simulink model "PubIfDecisionTOS_MDL"  (R2020b)
settings: configuration reference "DspaceConfig" (kept outside this file)
PostLoadFcn:
  | if any(exist('dsrtsu_mdlpostloadfcn', 'file') ~= 0), dsrtsu_mdlpostloadfcn('Execute', bdroot); end
InitFcn:
  | , if any(exist('dsmpb_private', 'file') ~= 0), dsmpb_private('dsmpb_mdlclblib', 'Init', bdroot); end,
undefined symbols (not defined in the file or in its folder): C_TOS_ACCEgoRAxletoFbumplength_m, C_TOS_ACCTargetFront_Flag, C_TOS_AEBJAPedObjDxThre_Val, C_TOS_AEBJAPedObjDyThre_Val, C_TOS_AEBJATargetSize_Val, C_TOS_AEBJAVehObjDxThre_Val, C_TOS_AEBJAVehObjDyThre_Val, C_TOS_AEBJuncPedTargetSize_Val, C_TOS_AEBLatObjDxThre_Val, C_TOS_AEBLatPedDyThre_Val, C_TOS_AEBLatTargetSize_Val, C_TOS_AEBLongTargetInEgoFront_Flag, C_TOS_axAbsGround_Parameter, C_TOS_CameraConfirmedFlag, C_TOS_CNsubjWidth, C_TOS_CurrentLaneCoreMinWidth_Val, C_TOS_CutInProb_Val_Zero, C_TOS_CutOutProb_Val_Zero, C_TOS_D2R_Val, C_TOS_DefaultValueObjectToCenterLine_dy, C_TOS_EgoCarWidth_Val, C_TOS_EgoDxRefPoint_m, C_TOS_EgoRAxletoFbumplength_m, C_TOS_HalfWidthVehicle_Con, C_TOS_HWA_CurrentLaneFlag, C_TOS_HWA_LeftLaneFlag, C_TOS_HWA_MovingDir_Vaild, C_TOS_HWA_MovState_Vaild, C_TOS_HWA_RightLaneFlag, C_TOS_LaneLineCourseErrorFront, C_TOS_LaneLineCourseErrorRear, C_TOS_MotorbikeDefaultWidth_m, C_TOS_NumberOfEffectiveTargets, C_TOS_Obj_Age_Val, C_TOS_Objdx_Constraint_Val, C_TOS_ObjectDefaultWidth_m, C_TOS_ObjInCurrentLane_Val, C_TOS_ObjInCurrentLaneValid, C_TOS_ObjInLeftLaneValid, C_TOS_ObjInRightLaneValid, C_TOS_ObjNotInCurrentLane_Val, C_TOS_ObjNotREElementType, C_TOS_ObjPredictDis_dy_ConstantVal_Zeros, C_TOS_ObjToCenterLine_ConstantVal_Zeros, C_TOS_OFMObjIDInvilad_Val, C_TOS_PIL_LatDisCons_Val_zero, C_TOS_PIL_ObjectCutInFlag_b, C_TOS_PIL_ObjectCutOutFlag_b, C_TOS_PIL_ObjLaneProb_al_Val, C_TOS_PP_ObjFusType_FC_Confirm_b, C_TOS_PP_ObjFusType_FC_FR_Confirm_b, C_TOS_PP_ObjFusType_FR_Confirm_b, C_TOS_RE_80BoolDefault_Val, C_TOS_RE_80Single181Default_Val, C_TOS_RE_80Single255Default_Val, C_TOS_RE_80Uint8Default_Val, C_TOS_RE_D2R, C_TOS_RE_D_180_Val, C_TOS_RE_InvalidObjectID_Val, C_TOS_RE_InvalidTargetChainDir_Val ... (+142)
libraries: simulink x1650, TOS_LIB x361, canfdmsglib x14
(part 40 of 69)

== system PubIfDecisionTOS_MDL/TOS_20201112/TOS_2012080320/TOS/LC_LCKie_ELK/TOS_HWA/CurrentLane/HWA_CurrentLane_Target/HWA_CLF_Target_3/HWA_CLR_Target_Default ==
  Action Port : ActionPort  ActionPortLabel=if(u1 ~= 0)
  Constant{1..4,7,12} (6 alike) : Constant  Value=0  OutDataTypeStr=boolean
  HWA_CLR_Target_3_TargeConfirm : Outport
  HWA_CLR_Target_3_MovState_ObserVale : Outport  Port=2
  HWA_CLR_Target_3_ObjType_ObserVale : Outport  Port=3
  HWA_CLR_Target_3_InCurrentLane_Flag_ObserVale : Outport  Port=4
  HWA_CLR_Target_3_TargetMovingDir_ObserVale : Outport  Port=5
  HWA_CLR_Target_3_DyConfirm_ObserVale : Outport  Port=6
  wires:
  Constant4/1 -> HWA_CLR_Target_3_TargeConfirm/1
  Constant1/1 -> HWA_CLR_Target_3_MovState_ObserVale/1
  Constant3/1 -> HWA_CLR_Target_3_ObjType_ObserVale/1
  Constant2/1 -> HWA_CLR_Target_3_InCurrentLane_Flag_ObserVale/1
  Constant12/1 -> HWA_CLR_Target_3_DyConfirm_ObserVale/1
  Constant7/1 -> HWA_CLR_Target_3_TargetMovingDir_ObserVale/1

== system PubIfDecisionTOS_MDL/TOS_20201112/TOS_2012080320/TOS/LC_LCKie_ELK/TOS_HWA/CurrentLane/HWA_Object_PreConfirm/TOS_HWA_CurrentLaneFront_TargPreConfirm/Default ==
  Action Port : ActionPort  ActionPortLabel=else
  Constant{1..10} (10 alike) : Constant  Value=0  OutDataTypeStr=boolean
  TOS_HWA_TargetPre_Filt_Flag : Outport
  TOS_HWA_TargetPre_1_ConditionFlag_ObserVale : Outport  Port=2
  TOS_HWA_TargetPre_FusionTypeFlag_ObserVale : Outport  Port=3
  TOS_HWA_TargetPre_PassedbyTarget_Flag_ObserVale : Outport  Port=4
  TOS_HWA_TargetPre_FenceFlag_ObserVale : Outport  Port=5
  TOS_HWA_TargetPre_ObjType_ObserVale : Outport  Port=6
  TOS_HWA_TargetPre_OverlapThre_Val_ObserVale : Outport  Port=7
  TOS_HWA_TargetPre_SameLane_Flag : Outport  Port=8
  TOS_HWA_TargetPre_2_OverlapThre_ObserVale : Outport  Port=9
  TOS_HWA_TargetPre_3_SameLane_Flag_ObserVale : Outport  Port=10
  wires:
  Constant2/1 -> TOS_HWA_TargetPre_Filt_Flag/1
  Constant9/1 -> TOS_HWA_TargetPre_3_SameLane_Flag_ObserVale/1
  Constant1/1 -> TOS_HWA_TargetPre_1_ConditionFlag_ObserVale/1
  Constant3/1 -> TOS_HWA_TargetPre_FusionTypeFlag_ObserVale/1
  Constant4/1 -> TOS_HWA_TargetPre_PassedbyTarget_Flag_ObserVale/1
  Constant5/1 -> TOS_HWA_TargetPre_FenceFlag_ObserVale/1
  Constant6/1 -> TOS_HWA_TargetPre_ObjType_ObserVale/1
  Constant7/1 -> TOS_HWA_TargetPre_OverlapThre_Val_ObserVale/1
  Constant8/1 -> TOS_HWA_TargetPre_SameLane_Flag/1
  Constant10/1 -> TOS_HWA_TargetPre_2_OverlapThre_ObserVale/1

== system PubIfDecisionTOS_MDL/TOS_20201112/TOS_2012080320/TOS/LC_LCKie_ELK/TOS_HWA/CurrentLane/HWA_Object_PreConfirm/TOS_HWA_CurrentLaneFront_TargPreConfirm/TOS_HWA_CurrentLaneFront_TargPreConfirm ==
  note: 行人、自行车目标过滤
  note: 判断是否为护栏目标
  note: 针对，选中目标后，过滤突然出现的纵向距离更近的单雷达静止目标
  Object_ID : Inport
  PP_ObjFusType_FC_FR_Confirm : Inport  Port=2
  PP_ObjFusType_FR_Confirm : Inport  Port=3
  PP_ObjFusType_FC_Confirm : Inport  Port=4
  Obj_MovingState : Inport  Port=5
  Obj_Dx : Inport  Port=6
  Object_ObstacleProb : Inport  Port=7
  Object_DY : Inport  Port=8
  Object_ObjType : Inport  Port=9
  TOS_TLJ_SameLaneConfirm_Flag : Inport  Port=10
  LM_LR_Line04_fCamValid : Inport  Port=11
  LM_LR_Line05_fCamValid : Inport  Port=12
  LM_LR_Line06_fCamValid : Inport  Port=13
  TOS_HWA_ID_K1 : Inport  Port=14
  TOS_HWA_Dx_K1 : Inport  Port=15
  PIL_OverlapRatio : Inport  Port=16
  PIL_OverlapRatio_K1 : Inport  Port=17
  PIL_OverlapRatio_K2 : Inport  Port=18
  LM_LR_Line04_dDisStart : Inport  Port=19
  LM_LR_Line04_dDisEnd : Inport  Port=20
  LM_LR_Line05_dDisStart : Inport  Port=21
  LM_LR_Line05_dDisEnd : Inport  Port=22
  LM_LR_Line06_dDisStart : Inport  Port=23
  LM_LR_Line06_dDisEnd : Inport  Port=24
  Action Port : ActionPort  ActionPortLabel=if(u1 == 1)
  " " : Subsystem
  Bus Creator : BusCreator  Inputs=24
  Bus Selector1 : BusSelector  OutputSignals=PP_ObjFusType_FR_Confirm,Obj_MovingState,Obj_Dx,TOS_HWA_ID_K1,TOS_HWA_Dx_K1,Object_ID
  Bus Selector2 : BusSelector  OutputSignals=PP_ObjFusType_FC_FR_Confirm,PP_ObjFusType_FC_Confirm,PP_ObjFusType_FR_Confirm
  Bus Selector3 : BusSelector  OutputSignals=PP_ObjFusType_FR_Confirm,Obj_MovingState,Object_ObstacleProb,Object_DY
  Bus Selector4 : BusSelector  OutputSignals=Obj_MovingState,Object_ObjType
  Bus Selector6 : BusSelector  OutputSignals=TOS_TLJ_SameLaneConfirm_Flag
  Compare To Constant2 : simulink/Logic and Bit Operations/Compare To Constant  relop===  const=C_TOS_ACCTargetFront_Flag  OutDataTypeStr=boolean
      settings: AttributesFormatString=C_TOS_ACCTargetFront_Flag = 1
  Logical Operator : Logic  Operator=NOT  AllPortsSameDT=off  OutDataTypeStr=boolean
  Logical Operator1 : Logic  Inputs=5  AllPortsSameDT=off  OutDataTypeStr=boolean
  Logical Operator2 : Logic  Operator=NOT  AllPortsSameDT=off  OutDataTypeStr=boolean
  Logical Operator3 : Logic  Operator=OR  AllPortsSameDT=off  OutDataTypeStr=boolean
  Overlap : Subsystem
  Subsystem : Subsystem
  Subsystem1 : Subsystem
  Subsystem3 : Subsystem
  TOS_HWA_DyConfirm : Subsystem
  TOS_HWA_TargetPre_Filt_Flag : Outport
  TOS_HWA_TargetPre_1_ConditionFlag_ObserVale : Outport  Port=2
  TOS_HWA_TargetPre_FusionTypeFlag_ObserVale : Outport  Port=3
  TOS_HWA_TargetPre_PassedbyTarget_Flag_ObserVale : Outport  Port=4
  TOS_HWA_TargetPre_FenceFlag_ObserVale : Outport  Port=5
  TOS_HWA_TargetPre_ObjType_ObserVale : Outport  Port=6
  TOS_HWA_TargetPre_OverlapThre_Val_ObserVale : Outport  Port=7
  TOS_HWA_TargetPre_SameLane_Flag : Outport  Port=8
  TOS_HWA_TargetPre_2_OverlapThre_ObserVale : Outport  Port=9
  TOS_HWA_TargetPre_3_SameLane_Flag_ObserVale : Outport  Port=10
  wires:
  Subsystem/1(TOS_HWA_TargetPre_TargetFusionTypeFlag) -> [TOS_HWA_TargetPre_FusionTypeFlag_ObserVale], Logical Operator1/1
  Subsystem1/1(TOS_HWA_TargetPre_ObjectPassedbyTarget_Flag) -> Logical Operator/1
  Subsystem3/1(TOS_HWA_TargetPre_FenceFlag) -> Logical Operator2/1
  Logical Operator2/1 -> [TOS_HWA_TargetPre_FenceFlag_ObserVale], Logical Operator1/3
  Logical Operator/1 -> [TOS_HWA_TargetPre_PassedbyTarget_Flag_ObserVale], Logical Operator1/2
  Bus Selector1/6 -> Subsystem1/6(Object_ID)  "<Object_ID>"
  PP_ObjFusType_FR_Confirm/1 -> Bus Creator/3  "PP_ObjFusType_FR_Confirm"
  Bus Selector1/4 -> Subsystem1/4(TOS_HWA_ID_K1)  "<TOS_HWA_ID_K1>"
  Object_ID/1 -> Bus Creator/1  "Object_ID"
  PP_ObjFusType_FC_Confirm/1 -> Bus Creator/4  "PP_ObjFusType_FC_Confirm"
  Bus Selector2/1 -> Subsystem/1(PP_ObjFusType_FC_FR_Confirm)  "<PP_ObjFusType_FC_FR_Confirm>"
  Bus Selector2/3 -> Subsystem/3(PP_ObjFusType_FC_Confirm)  "<PP_ObjFusType_FR_Confirm>"
  Bus Selector1/1 -> Subsystem1/1(FR_Confirm)  "<PP_ObjFusType_FR_Confirm>"
  Bus Selector2/2 -> Subsystem/2(PP_ObjFusType_FR_Confirm)  "<PP_ObjFusType_FC_Confirm>"
  Bus Selector1/5 -> Subsystem1/5(TOS_HWA_Dx_K1)  "<TOS_HWA_Dx_K1>"
  PP_ObjFusType_FC_FR_Confirm/1 -> Bus Creator/2  "PP_ObjFusType_FC_FR_Confirm"
  TOS_HWA_ID_K1/1 -> Bus Creator/14  "TOS_HWA_ID_K1"
  Object_DY/1 -> Bus Creator/8  "Object_DY"
  Bus Selector1/2 -> Subsystem1/2(Obj_MovingState)  "<Obj_MovingState>"
  Bus Selector3/2 -> Subsystem3/2(Obj_MovingState)  "<Obj_MovingState>"
  TOS_HWA_Dx_K1/1 -> Bus Creator/15  "TOS_HWA_Dx_K1"
  Obj_MovingState/1 -> Bus Creator/5  "Obj_MovingState"
  Bus Selector1/3 -> Subsystem1/3(Obj_Dx)  "<Obj_Dx>"
  Object_ObstacleProb/1 -> Bus Creator/7  "Object_ObstacleProb"
  Bus Selector3/3 -> Subsystem3/3(Object_ObstacleProb)  "<Object_ObstacleProb>"
  Bus Selector3/4 -> Subsystem3/4(Object_DY)  "<Object_DY>"
  Bus Selector3/1 -> Subsystem3/1(FR_Confirm)  "<PP_ObjFusType_FR_Confirm>"
  Obj_Dx/1 -> Bus Creator/6  "Obj_Dx"
  Bus Selector4/2 -> " "/2(Object_Type)  "<Object_ObjType>"
  Bus Selector4/1 -> " "/1(object_MovingState)  "<Obj_MovingState>"
  " "/1(TOS_HWA_ObjType) -> [TOS_HWA_TargetPre_ObjType_ObserVale], Logical Operator1/4
  Object_ObjType/1 -> Bus Creator/9  "Object_ObjType"
  [TOS_HWA_TargetPre_FusionTypeFlag_ObserVale] -> TOS_HWA_TargetPre_FusionTypeFlag_ObserVale/1
  [TOS_HWA_TargetPre_PassedbyTarget_Flag_ObserVale] -> TOS_HWA_TargetPre_PassedbyTarget_Flag_ObserVale/1
  [TOS_HWA_TargetPre_FenceFlag_ObserVale] -> TOS_HWA_TargetPre_FenceFlag_ObserVale/1
  [TOS_HWA_TargetPre_ObjType_ObserVale] -> TOS_HWA_TargetPre_ObjType_ObserVale/1
  PIL_OverlapRatio/1 -> Bus Creator/16  "PIL_OverlapRatio"
  TOS_HWA_DyConfirm/1(TOS_HWA_DyConfirm) -> [TOS_HWA_TargetPre_OverlapThre_Val_ObserVale], Logical Operator1/5
  [TOS_HWA_TargetPre_OverlapThre_Val_ObserVale] -> TOS_HWA_TargetPre_OverlapThre_Val_ObserVale/1
  TOS_TLJ_SameLaneConfirm_Flag/1 -> Bus Creator/10  "TOS_TLJ_SameLaneConfirm_Flag"
  Bus Selector6/1 -> Compare To Constant2/1  "<TOS_TLJ_SameLaneConfirm_Flag>"
  Compare To Constant2/1 -> [TOS_HWA_TargetPre_3_SameLane_Flag_ObserVale], Logical Operator3/2
  Logical Operator3/1 -> TOS_HWA_TargetPre_SameLane_Flag/1
  Logical Operator1/1 -> [TOS_HWA_TargetPre_1_ConditionFlag_ObserVale], TOS_HWA_TargetPre_Filt_Flag/1
  [TOS_HWA_TargetPre_2_OverlapThre_ObserVale] -> TOS_HWA_TargetPre_2_OverlapThre_ObserVale/1
  [TOS_HWA_TargetPre_3_SameLane_Flag_ObserVale] -> TOS_HWA_TargetPre_3_SameLane_Flag_ObserVale/1
  [TOS_HWA_TargetPre_1_ConditionFlag_ObserVale] -> TOS_HWA_TargetPre_1_ConditionFlag_ObserVale/1
  PIL_OverlapRatio_K1/1 -> Bus Creator/17  "PIL_OverlapRatio_K1"
  PIL_OverlapRatio_K2/1 -> Bus Creator/18  "PIL_OverlapRatio_K2"
  LM_LR_Line04_fCamValid/1 -> Bus Creator/11  "LM_LR_Line04_fCamValid"
  LM_LR_Line05_fCamValid/1 -> Bus Creator/12  "LM_LR_Line05_fCamValid"
  LM_LR_Line06_fCamValid/1 -> Bus Creator/13  "LM_LR_Line06_fCamValid"
  LM_LR_Line04_dDisStart/1 -> Bus Creator/19  "LM_LR_Line04_dDisStart"
  LM_LR_Line04_dDisEnd/1 -> Bus Creator/20  "LM_LR_Line04_dDisEnd"
  LM_LR_Line05_dDisStart/1 -> Bus Creator/21  "LM_LR_Line05_dDisStart"
  LM_LR_Line05_dDisEnd/1 -> Bus Creator/22  "LM_LR_Line05_dDisEnd"
  LM_LR_Line06_dDisStart/1 -> Bus Creator/23  "LM_LR_Line06_dDisStart"
  LM_LR_Line06_dDisEnd/1 -> Bus Creator/24  "LM_LR_Line06_dDisEnd"
  Bus Creator/1 -> Bus Selector6/1, Overlap/1(LM), TOS_HWA_DyConfirm/1(TOS_HWA_Dy), Bus Selector4/1, Bus Selector3/1, Bus Selector1/1, Bus Selector2/1
  Overlap/1(Overlap) -> [TOS_HWA_TargetPre_2_OverlapThre_ObserVale], Logical Operator3/1

== system PubIfDecisionTOS_MDL/TOS_20201112/TOS_2012080320/TOS/LC_LCKie_ELK/TOS_HWA/CurrentLane/HWA_Object_PreConfirm/TOS_HWA_CurrentLaneFront_TargPreConfirm/TOS_HWA_CurrentLaneRear_TargPreConfirmDefault ==
  Action Port : ActionPort  ActionPortLabel=elseif(u2 == 1)
  Constant{1..10} (10 alike) : Constant  OutDataTypeStr=boolean
  TOS_HWA_TargetPre_Filt_Flag : Outport
  TOS_HWA_TargetPre_1_ConditionFlag_ObserVale : Outport  Port=2
  TOS_HWA_TargetPre_FusionTypeFlag_ObserVale : Outport  Port=3
  TOS_HWA_TargetPre_PassedbyTarget_Flag_ObserVale : Outport  Port=4
  TOS_HWA_TargetPre_FenceFlag_ObserVale : Outport  Port=5
  TOS_HWA_TargetPre_ObjType_ObserVale : Outport  Port=6
  TOS_HWA_TargetPre_OverlapThre_Val_ObserVale : Outport  Port=7
  TOS_HWA_TargetPre_SameLane_Flag : Outport  Port=8
  TOS_HWA_TargetPre_2_OverlapThre_ObserVale : Outport  Port=9
  TOS_HWA_TargetPre_3_SameLane_Flag_ObserVale : Outport  Port=10
  wires:
  Constant10/1 -> TOS_HWA_TargetPre_2_OverlapThre_ObserVale/1
  Constant8/1 -> TOS_HWA_TargetPre_SameLane_Flag/1
  Constant7/1 -> TOS_HWA_TargetPre_OverlapThre_Val_ObserVale/1
  Constant6/1 -> TOS_HWA_TargetPre_ObjType_ObserVale/1
  Constant5/1 -> TOS_HWA_TargetPre_FenceFlag_ObserVale/1
  Constant4/1 -> TOS_HWA_TargetPre_PassedbyTarget_Flag_ObserVale/1
  Constant3/1 -> TOS_HWA_TargetPre_FusionTypeFlag_ObserVale/1
  Constant1/1 -> TOS_HWA_TargetPre_1_ConditionFlag_ObserVale/1
  Constant9/1 -> TOS_HWA_TargetPre_3_SameLane_Flag_ObserVale/1
  Constant2/1 -> TOS_HWA_TargetPre_Filt_Flag/1

== system PubIfDecisionTOS_MDL/TOS_20201112/TOS_2012080320/TOS/LC_LCKie_ELK/TOS_HWA/LeftLane/HWA_Object_PreConfirm/HWA_Object_PreConfirm/Default ==
  Action Port : ActionPort  ActionPortLabel=else
  Constant{2,5..6,8,10} (5 alike) : Constant  Value=0  OutDataTypeStr=boolean
  TOS_HWA_TargetPre_Confirm_Filt_Flag : Outport
  TOS_HWA_TargetPre_FusionTypeFlag_ObserVale : Outport  Port=2
  TOS_HWA_TargetPre_PassedbyTarget_Flag_ObserVale : Outport  Port=3
  TOS_HWA_TargetPre_ObjType_ObserVale : Outport  Port=4
  TOS_HWA_DyConfirm_ObserVale : Outport  Port=5
  wires:
  Constant2/1 -> TOS_HWA_TargetPre_Confirm_Filt_Flag/1
  Constant5/1 -> TOS_HWA_TargetPre_FusionTypeFlag_ObserVale/1
  Constant6/1 -> TOS_HWA_TargetPre_PassedbyTarget_Flag_ObserVale/1
  Constant8/1 -> TOS_HWA_TargetPre_ObjType_ObserVale/1
  Constant10/1 -> TOS_HWA_DyConfirm_ObserVale/1

== system PubIfDecisionTOS_MDL/TOS_20201112/TOS_2012080320/TOS/LC_LCKie_ELK/TOS_HWA/LeftLane/HWA_Object_PreConfirm/HWA_Object_PreConfirm/HWA_Object_PreConfirm ==
  Object_ID : Inport
  PP_ObjFusType_FC_FR_Confirm : Inport  Port=2
  PP_ObjFusType_FR_Confirm : Inport  Port=3
  PP_ObjFusType_FC_Confirm : Inport  Port=4
  Obj_MovingState : Inport  Port=5
  Obj_Dx : Inport  Port=6
  Object_ObstacleProb : Inport  Port=7
  Object_DY : Inport  Port=8
  Object_ObjType : Inport  Port=9
  Action Port : ActionPort  ActionPortLabel=if(u1 == 1)
  " " : Subsystem
  Bus Creator : BusCreator  Inputs=9
  Bus Selector1 : BusSelector  OutputSignals=PP_ObjFusType_FC_Confirm,Obj_MovingState
  Bus Selector2 : BusSelector  OutputSignals=PP_ObjFusType_FC_FR_Confirm,PP_ObjFusType_FC_Confirm,PP_ObjFusType_FR_Confirm
  Bus Selector4 : BusSelector  OutputSignals=Object_ObjType
  Constant1 : Constant  OutDataTypeStr=boolean
  Logical Operator1 : Logic  Inputs=4  AllPortsSameDT=off  OutDataTypeStr=boolean
  Subsystem : Subsystem
  Subsystem1 : Subsystem
  TOS_HWA_DyConfirm : Subsystem
  Terminator : Terminator
  TOS_HWA_TargetPre_Confirm_Filt_Flag : Outport
  TOS_HWA_TargetPre_FusionTypeFlag_ObserVale : Outport  Port=2
  TOS_HWA_TargetPre_PassedbyTarget_Flag_ObserVale : Outport  Port=3
  TOS_HWA_TargetPre_ObjType_ObserVale : Outport  Port=4
  TOS_HWA_DyConfirm_ObserVale : Outport  Port=5
  wires:
  Subsystem/1(TOS_HWA_TargetPre_TargetFusionTypeFlag) -> [TOS_HWA_TargetPre_FusionTypeFlag_ObserVale], Logical Operator1/1
  Subsystem1/1(TOS_HWA_TargetPre_ObjectPassedbyTarget_Flag) -> [TOS_HWA_TargetPre_PassedbyTarget_Flag_ObserVale], Logical Operator1/2
  PP_ObjFusType_FR_Confirm/1 -> Bus Creator/3  "PP_ObjFusType_FR_Confirm"
  Object_ID/1 -> Bus Creator/1  "Object_ID"
  PP_ObjFusType_FC_Confirm/1 -> Bus Creator/4  "PP_ObjFusType_FC_Confirm"
  Bus Selector2/1 -> Subsystem/1(PP_ObjFusType_FC_FR_Confirm)  "<PP_ObjFusType_FC_FR_Confirm>"
  Bus Selector2/3 -> Subsystem/3(PP_ObjFusType_FC_Confirm)  "<PP_ObjFusType_FR_Confirm>"
  Bus Selector1/1 -> Subsystem1/1(PP_ObjFusType_FC_Confirm)  "<PP_ObjFusType_FC_Confirm>"
  Bus Selector2/2 -> Subsystem/2(PP_ObjFusType_FR_Confirm)  "<PP_ObjFusType_FC_Confirm>"
  PP_ObjFusType_FC_FR_Confirm/1 -> Bus Creator/2  "PP_ObjFusType_FC_FR_Confirm"
  Object_DY/1 -> Bus Creator/8  "Object_DY"
  Bus Selector1/2 -> Subsystem1/2(Obj_MovingState)  "<Obj_MovingState>"
  Obj_MovingState/1 -> Bus Creator/5  "Obj_MovingState"
  Object_ObstacleProb/1 -> Bus Creator/7  "Object_ObstacleProb"
  Obj_Dx/1 -> Bus Creator/6  "Obj_Dx"
  Bus Selector4/1 -> " "/1(Object_Type)  "<Object_ObjType>"
  " "/1(TOS_HWA_TargetPre_ObjType) -> Logical Operator1/3, [TOS_HWA_TargetPre_ObjType_ObserVale]
  Object_ObjType/1 -> Bus Creator/9  "Object_ObjType"
  [TOS_HWA_TargetPre_FusionTypeFlag_ObserVale] -> TOS_HWA_TargetPre_FusionTypeFlag_ObserVale/1
  [TOS_HWA_TargetPre_PassedbyTarget_Flag_ObserVale] -> TOS_HWA_TargetPre_PassedbyTarget_Flag_ObserVale/1
  [TOS_HWA_TargetPre_ObjType_ObserVale] -> TOS_HWA_TargetPre_ObjType_ObserVale/1
  Constant1/1 -> Logical Operator1/4, [TOS_HWA_DyConfirm_ObserVale]
  [TOS_HWA_DyConfirm_ObserVale] -> TOS_HWA_DyConfirm_ObserVale/1
  Logical Operator1/1 -> TOS_HWA_TargetPre_Confirm_Filt_Flag/1
  Bus Creator/1 -> TOS_HWA_DyConfirm/1(TOS_HWA_Dy), Bus Selector4/1, Bus Selector1/1, Bus Selector2/1
  TOS_HWA_DyConfirm/1(TOS_HWA_TargetPre_DyConfirm) -> Terminator/1

== system PubIfDecisionTOS_MDL/TOS_20201112/TOS_2012080320/TOS/LC_LCKie_ELK/TOS_HWA/LeftLane/HWA_Object_PreConfirm/HWA_Object_PreConfirm/HWA_Object_PreConfirmDefault1 ==
  Action Port : ActionPort  ActionPortLabel=elseif(u2 == 1)
  Constant{1..5} (5 alike) : Constant  OutDataTypeStr=boolean
  TOS_HWA_TargetPre_Confirm_Filt_Flag : Outport
  TOS_HWA_TargetPre_FusionTypeFlag_ObserVale : Outport  Port=2
  TOS_HWA_TargetPre_PassedbyTarget_Flag_ObserVale : Outport  Port=3
  TOS_HWA_TargetPre_ObjType_ObserVale : Outport  Port=4
  TOS_HWA_DyConfirm_ObserVale : Outport  Port=5
  wires:
  Constant5/1 -> TOS_HWA_DyConfirm_ObserVale/1
  Constant3/1 -> TOS_HWA_TargetPre_ObjType_ObserVale/1
  Constant4/1 -> TOS_HWA_TargetPre_PassedbyTarget_Flag_ObserVale/1
  Constant1/1 -> TOS_HWA_TargetPre_FusionTypeFlag_ObserVale/1
  Constant2/1 -> TOS_HWA_TargetPre_Confirm_Filt_Flag/1

== system PubIfDecisionTOS_MDL/TOS_20201112/TOS_2012080320/TOS/LC_LCKie_ELK/TOS_HWA/LeftLane/TOS_HWA_LeftLane/TOS_HWA_LeftLane/TOS_HWA ==
  HWA_LeftLane_ObjIndex : Inport
  PP_ObjMovingDirSignalProcessing : Inport  Port=2
  Object_VX : Inport  Port=3
  Object_VY : Inport  Port=4
  Object_Type : Inport  Port=5
  object_MovingState : Inport  Port=6
  TOS_TLJ_LeftLaneConfirm_Flag : Inport  Port=7
  Object_DX : Inport  Port=8
  Object_DY : Inport  Port=9
  Object_Fus_Type : Inport  Port=10
  Object_HeadingAngle : Inport  Port=11
  PP_ObjFusType_FC_FR_Confirm : Inport  Port=12
  PP_ObjFusType_FR_Confirm : Inport  Port=13
  PP_ObjFusType_FC_Confirm : Inport  Port=14
  VIE_EgoVelocity : Inport  Port=15
  Action Port : ActionPort  ActionPortLabel=else
  HWA_LeftLane : Subsystem
  Selector{,1..12} (13 alike) : Selector  InputPortWidth=80  IndexOptions=Index vector (port)  Indices=[1 3]  OutputSizes=1
  TOS_HWA_TargetInLeftLane_b : Outport
  TOS_HWA_LeftFront_TargConfirm_b : Outport  Port=2
  TOS_HWA_LeftRear_TargConfirm_b : Outport  Port=3
  TOS_HWA_LeftFront_FusType_ObserVale : Outport  Port=4
  TOS_HWA_InLeftLane_Front_Flag_ObserVale : Outport  Port=5
  TOS_HWA_LeftFront_TargMovDir_ObserVale : Outport  Port=6
  TOS_HWA_LeftRear_MovState_ObserVale : Outport  Port=7
  TOS_HWA_LeftRear_FusionType_ObserVale : Outport  Port=8
  TOS_HWA_InLeftLane_Rear_Flag_ObserVale : Outport  Port=9
  TOS_HWA_LeftRear_TargetMovingDir_ObserVale : Outport  Port=10
  TOS_HWA_LeftRear_DyConfirm_ObserVale : Outport  Port=11
  wires:
  Selector12/1 -> HWA_LeftLane/9(Object_DY)
  Object_DY/1 -> Selector12/1  "Object_DX"
  HWA_LeftLane_ObjIndex/1 -> Selector2/2, Selector3/2, Selector4/2, Selector5/2, Selector6/2, Selector7/2, Selector8/2, Selector9/2, Selector10/2, Selector11/2, Selector12/2, Selector1/2, Selector/2  "HWA_LeftLane_ObjIndex"
  Object_HeadingAngle/1 -> Selector4/1  "Object_HeadingAngle"
  PP_ObjMovingDirSignalProcessing/1 -> Selector3/1  "PP_ObjMovingDirSignalProcessing"
  Object_VX/1 -> Selector/1  "Object_VX"
  Object_VY/1 -> Selector1/1  "Object_VY"
  Object_Type/1 -> Selector5/1  "Object_Type"
  TOS_TLJ_LeftLaneConfirm_Flag/1 -> Selector6/1  "TOS_TLJ_LeftLaneConfirm_Flag"
  Object_DX/1 -> Selector7/1  "Object_DX"
  Object_Fus_Type/1 -> Selector8/1  "Object_Fus_Type"
  PP_ObjFusType_FC_FR_Confirm/1 -> Selector9/1  "PP_ObjFusType_FC_FR_Confirm"
  PP_ObjFusType_FR_Confirm/1 -> Selector10/1  "PP_ObjFusType_FR_Confirm"
  PP_ObjFusType_FC_Confirm/1 -> Selector11/1  "PP_ObjFusType_FC_Confirm"
  object_MovingState/1 -> Selector2/1  "object_MovingState"
  Selector11/1 -> HWA_LeftLane/13(PP_ObjFusType_FC_Confirm)
  Selector10/1 -> HWA_LeftLane/12(PP_ObjFusType_FR_Confirm)
  Selector9/1 -> HWA_LeftLane/11(PP_ObjFusType_FC_FR_Confirm)
  Selector8/1 -> HWA_LeftLane/10(Object_Fus_Type)
  Selector7/1 -> HWA_LeftLane/8(Object_DX)
  Selector6/1 -> HWA_LeftLane/7(TOS_TLJ_LeftLaneConfirm_Flag)
  Selector5/1 -> HWA_LeftLane/6(Object_Type)
  Selector4/1 -> HWA_LeftLane/5(Object_HeadingAngle)
  Selector3/1 -> HWA_LeftLane/4(PP_ObjMovingDirSignalProcessing)
  Selector2/1 -> HWA_LeftLane/3(object_MovingState)
  Selector1/1 -> HWA_LeftLane/2(Object_VY)
  Selector/1 -> HWA_LeftLane/1(Object_VX)
  VIE_EgoVelocity/1 -> HWA_LeftLane/14(VIE_EgoVelocity)  "VIE_EgoVelocity"
  HWA_LeftLane/1(TOS_HWA_TargetInLeftLane_b) -> TOS_HWA_TargetInLeftLane_b/1
  HWA_LeftLane/2(TOS_HWA_LeftFront_TargConfirm_b) -> TOS_HWA_LeftFront_TargConfirm_b/1
  HWA_LeftLane/3(TOS_HWA_LeftRear_TargConfirm_b) -> TOS_HWA_LeftRear_TargConfirm_b/1
  HWA_LeftLane/4(TOS_HWA_LeftFront_FusType_ObserVale) -> TOS_HWA_LeftFront_FusType_ObserVale/1
  HWA_LeftLane/5(TOS_HWA_InLeftLane_Front_Flag_ObserVale) -> TOS_HWA_InLeftLane_Front_Flag_ObserVale/1
  HWA_LeftLane/6(TOS_HWA_LeftFront_TargMovDir_ObserVale) -> TOS_HWA_LeftFront_TargMovDir_ObserVale/1
  HWA_LeftLane/7(TOS_HWA_LeftRear_MovState_ObserVale) -> TOS_HWA_LeftRear_MovState_ObserVale/1
  HWA_LeftLane/8(TOS_HWA_LeftRear_FusionType_ObserVale) -> TOS_HWA_LeftRear_FusionType_ObserVale/1
  HWA_LeftLane/9(TOS_HWA_InLeftLane_Rear_Flag_ObserVale) -> TOS_HWA_InLeftLane_Rear_Flag_ObserVale/1
  HWA_LeftLane/10(TOS_HWA_LeftRear_TargetMovingDir_ObserVale) -> TOS_HWA_LeftRear_TargetMovingDir_ObserVale/1
  HWA_LeftLane/11(TOS_HWA_LeftRear_DyConfirm_ObserVale) -> TOS_HWA_LeftRear_DyConfirm_ObserVale/1

== system PubIfDecisionTOS_MDL/TOS_20201112/TOS_2012080320/TOS/LC_LCKie_ELK/TOS_HWA/LeftLane/TOS_HWA_LeftLane/TOS_HWA_LeftLane/TOS_HWA_Default ==
  Action Port : ActionPort  ActionPortLabel=if(u1 ~= 0)
  Constant{1..11} (11 alike) : Constant  Value=0  OutDataTypeStr=boolean
  TOS_HWA_TargetInLeftLane_b : Outport
  TOS_HWA_LeftFront_TargConfirm_b : Outport  Port=2
  TOS_HWA_LeftRear_TargConfirm_b : Outport  Port=3
  TOS_HWA_LeftFront_FusType_ObserVale : Outport  Port=4
  TOS_HWA_InLeftLane_Front_Flag_ObserVale : Outport  Port=5
  TOS_HWA_LeftFront_TargMovDir_ObserVale : Outport  Port=6
  TOS_HWA_LeftRear_MovState_ObserVale : Outport  Port=7
  TOS_HWA_LeftRear_FusionType_ObserVale : Outport  Port=8
  TOS_HWA_InLeftLane_Rear_Flag_ObserVale : Outport  Port=9
  TOS_HWA_LeftRear_TargetMovingDir_ObserVale : Outport  Port=10
  TOS_HWA_LeftRear_DyConfirm_ObserVale : Outport  Port=11
  wires:
  Constant11/1 -> TOS_HWA_LeftRear_TargetMovingDir_ObserVale/1
  Constant10/1 -> TOS_HWA_LeftRear_DyConfirm_ObserVale/1
  Constant9/1 -> TOS_HWA_InLeftLane_Rear_Flag_ObserVale/1
  Constant8/1 -> TOS_HWA_InLeftLane_Front_Flag_ObserVale/1
  Constant5/1 -> TOS_HWA_LeftFront_TargMovDir_ObserVale/1
  Constant6/1 -> TOS_HWA_LeftRear_FusionType_ObserVale/1
  Constant7/1 -> TOS_HWA_LeftRear_MovState_ObserVale/1
  Constant3/1 -> TOS_HWA_LeftRear_TargConfirm_b/1
  Constant2/1 -> TOS_HWA_LeftFront_FusType_ObserVale/1
  Constant1/1 -> TOS_HWA_LeftFront_TargConfirm_b/1
  Constant4/1 -> TOS_HWA_TargetInLeftLane_b/1

== system PubIfDecisionTOS_MDL/TOS_20201112/TOS_2012080320/TOS/LC_LCKie_ELK/TOS_HWA/RightLane/HWA_Object_PreConfirm/HWA_Object_PreConfirm/Default ==
  Action Port : ActionPort  ActionPortLabel=else
  Constant{2,5..6,8,10} (5 alike) : Constant  Value=0  OutDataTypeStr=boolean
  TOS_HWA_TargetPre_Confirm_Filt_Flag : Outport
  TOS_HWA_TargetPre_FusionTypeFlag_ObserVale : Outport  Port=2
  TOS_HWA_TargetPre_PassedbyTarget_Flag_ObserVale : Outport  Port=3
  TOS_HWA_TargetPre_ObjType_ObserVale : Outport  Port=4
  TOS_HWA_DyConfirm_ObserVale : Outport  Port=5
  wires:
  Constant2/1 -> TOS_HWA_TargetPre_Confirm_Filt_Flag/1
  Constant5/1 -> TOS_HWA_TargetPre_FusionTypeFlag_ObserVale/1
  Constant6/1 -> TOS_HWA_TargetPre_PassedbyTarget_Flag_ObserVale/1
  Constant8/1 -> TOS_HWA_TargetPre_ObjType_ObserVale/1
  Constant10/1 -> TOS_HWA_DyConfirm_ObserVale/1

== system PubIfDecisionTOS_MDL/TOS_20201112/TOS_2012080320/TOS/LC_LCKie_ELK/TOS_HWA/RightLane/HWA_Object_PreConfirm/HWA_Object_PreConfirm/HWA_Object_PreConfirm ==
  Object_ID : Inport
  PP_ObjFusType_FC_FR_Confirm : Inport  Port=2
  PP_ObjFusType_FR_Confirm : Inport  Port=3
  PP_ObjFusType_FC_Confirm : Inport  Port=4
  Obj_MovingState : Inport  Port=5
  Obj_Dx : Inport  Port=6
  Object_ObstacleProb : Inport  Port=7
  Object_DY : Inport  Port=8
  Object_ObjType : Inport  Port=9
  Action Port : ActionPort  ActionPortLabel=if(u1 == 1)
  " " : Subsystem
  Bus Creator : BusCreator  Inputs=9
  Bus Selector1 : BusSelector  OutputSignals=PP_ObjFusType_FC_Confirm,Obj_MovingState
  Bus Selector2 : BusSelector  OutputSignals=PP_ObjFusType_FC_FR_Confirm,PP_ObjFusType_FC_Confirm,PP_ObjFusType_FR_Confirm
  Bus Selector4 : BusSelector  OutputSignals=Object_ObjType
  Constant1 : Constant  OutDataTypeStr=boolean
  Logical Operator1 : Logic  Inputs=4  AllPortsSameDT=off  OutDataTypeStr=boolean
  Subsystem : Subsystem
  Subsystem1 : Subsystem
  TOS_HWA_DyConfirm : Subsystem
  Terminator : Terminator
  TOS_HWA_TargetPre_Confirm_Filt_Flag : Outport
  TOS_HWA_TargetPre_FusionTypeFlag_ObserVale : Outport  Port=2
  TOS_HWA_TargetPre_PassedbyTarget_Flag_ObserVale : Outport  Port=3
  TOS_HWA_TargetPre_ObjType_ObserVale : Outport  Port=4
  TOS_HWA_DyConfirm_ObserVale : Outport  Port=5
  wires:
  Subsystem/1(TOS_HWA_TargetPre_TargetFusionTypeFlag) -> [TOS_HWA_TargetPre_FusionTypeFlag_ObserVale], Logical Operator1/1
  Subsystem1/1(TOS_HWA_TargetPre_ObjectPassedbyTarget_Flag) -> [TOS_HWA_TargetPre_PassedbyTarget_Flag_ObserVale], Logical Operator1/2
  PP_ObjFusType_FR_Confirm/1 -> Bus Creator/3  "PP_ObjFusType_FR_Confirm"
  Object_ID/1 -> Bus Creator/1  "Object_ID"
  PP_ObjFusType_FC_Confirm/1 -> Bus Creator/4  "PP_ObjFusType_FC_Confirm"
  Bus Selector2/1 -> Subsystem/1(PP_ObjFusType_FC_FR_Confirm)  "<PP_ObjFusType_FC_FR_Confirm>"
  Bus Selector2/3 -> Subsystem/3(PP_ObjFusType_FC_Confirm)  "<PP_ObjFusType_FR_Confirm>"
  Bus Selector1/1 -> Subsystem1/1(PP_ObjFusType_FC_Confirm)  "<PP_ObjFusType_FC_Confirm>"
  Bus Selector2/2 -> Subsystem/2(PP_ObjFusType_FR_Confirm)  "<PP_ObjFusType_FC_Confirm>"
  PP_ObjFusType_FC_FR_Confirm/1 -> Bus Creator/2  "PP_ObjFusType_FC_FR_Confirm"
  Object_DY/1 -> Bus Creator/8  "Object_DY"
  Bus Selector1/2 -> Subsystem1/2(Obj_MovingState)  "<Obj_MovingState>"
  Obj_MovingState/1 -> Bus Creator/5  "Obj_MovingState"
  Object_ObstacleProb/1 -> Bus Creator/7  "Object_ObstacleProb"
  Obj_Dx/1 -> Bus Creator/6  "Obj_Dx"
  Bus Selector4/1 -> " "/1(Object_Type)  "<Object_ObjType>"
  " "/1(TOS_HWA_TargetPre_ObjType) -> Logical Operator1/3, [TOS_HWA_TargetPre_ObjType_ObserVale]
  Object_ObjType/1 -> Bus Creator/9  "Object_ObjType"
  [TOS_HWA_TargetPre_FusionTypeFlag_ObserVale] -> TOS_HWA_TargetPre_FusionTypeFlag_ObserVale/1
  [TOS_HWA_TargetPre_PassedbyTarget_Flag_ObserVale] -> TOS_HWA_TargetPre_PassedbyTarget_Flag_ObserVale/1
  [TOS_HWA_TargetPre_ObjType_ObserVale] -> TOS_HWA_TargetPre_ObjType_ObserVale/1
  Constant1/1 -> Logical Operator1/4, [TOS_HWA_DyConfirm_ObserVale]
  [TOS_HWA_DyConfirm_ObserVale] -> TOS_HWA_DyConfirm_ObserVale/1
  Logical Operator1/1 -> TOS_HWA_TargetPre_Confirm_Filt_Flag/1
  Bus Creator/1 -> TOS_HWA_DyConfirm/1(TOS_HWA_Dy), Bus Selector4/1, Bus Selector1/1, Bus Selector2/1
  TOS_HWA_DyConfirm/1(TOS_HWA_TargetPre_DyConfirm) -> Terminator/1

== system PubIfDecisionTOS_MDL/TOS_20201112/TOS_2012080320/TOS/LC_LCKie_ELK/TOS_HWA/RightLane/HWA_Object_PreConfirm/HWA_Object_PreConfirm/HWA_Object_PreConfirmDefault1 ==
  Action Port : ActionPort  ActionPortLabel=elseif(u2 == 1)
  Constant{1..5} (5 alike) : Constant  OutDataTypeStr=boolean
  TOS_HWA_TargetPre_Confirm_Filt_Flag : Outport
  TOS_HWA_TargetPre_FusionTypeFlag_ObserVale : Outport  Port=2
  TOS_HWA_TargetPre_PassedbyTarget_Flag_ObserVale : Outport  Port=3
  TOS_HWA_TargetPre_ObjType_ObserVale : Outport  Port=4
  TOS_HWA_DyConfirm_ObserVale : Outport  Port=5
  wires:
  Constant5/1 -> TOS_HWA_DyConfirm_ObserVale/1
  Constant3/1 -> TOS_HWA_TargetPre_ObjType_ObserVale/1
  Constant4/1 -> TOS_HWA_TargetPre_PassedbyTarget_Flag_ObserVale/1
  Constant1/1 -> TOS_HWA_TargetPre_FusionTypeFlag_ObserVale/1
  Constant2/1 -> TOS_HWA_TargetPre_Confirm_Filt_Flag/1

== system PubIfDecisionTOS_MDL/TOS_20201112/TOS_2012080320/TOS/LC_LCKie_ELK/TOS_HWA/RightLane/TOS_HWA_RightLane/TOS_HWA_RightLane/TOS_HWA ==
  HWA_RightLane_ObjIndex : Inport
  PP_ObjMovingDirSignalProcessing : Inport  Port=2
  Object_VX : Inport  Port=3
  Object_VY : Inport  Port=4
  Object_Type : Inport  Port=5
  object_MovingState : Inport  Port=6
  TOS_TLJ_RightLaneConfirm_Flag : Inport  Port=7
  Object_DX : Inport  Port=8
  Object_DY : Inport  Port=9
  Object_Fus_Type : Inport  Port=10
  Object_HeadingAngle : Inport  Port=11
  PP_ObjFusType_FC_FR_Confirm : Inport  Port=12
  PP_ObjFusType_FR_Confirm : Inport  Port=13
  PP_ObjFusType_FC_Confirm : Inport  Port=14
  VIE_EgoVelocity : Inport  Port=15
  Action Port : ActionPort  ActionPortLabel=else
  HWA_RightLane : Subsystem
  Selector{,1..12} (13 alike) : Selector  InputPortWidth=80  IndexOptions=Index vector (port)  Indices=[1 3]  OutputSizes=1
  TOS_HWA_TargetInRightLane_b : Outport
  TOS_HWA_RightFront_TargConfirm_b : Outport  Port=2
  TOS_HWA_RightRear_TargConfirm_b : Outport  Port=3
  TOS_HWA_RightFront_FusType_ObserVale : Outport  Port=4
  TOS_HWA_InRightLane_Front_Flag_ObserVale : Outport  Port=5
  TOS_HWA_RightFront_TargMovDir_ObserVale : Outport  Port=6
  TOS_HWA_RightRear_MovState_ObserVale : Outport  Port=7
  TOS_HWA_RightRear_FusionType_ObserVale : Outport  Port=8
  TOS_HWA_InRightLane_Rear_Flag_ObserVale : Outport  Port=9
  TOS_HWA_RightRear_TargetMovingDir_ObserVale : Outport  Port=10
  TOS_HWA_RightRear_DyConfirm_ObserVale : Outport  Port=11
  wires:
  VIE_EgoVelocity/1 -> HWA_RightLane/14(VIE_EgoVelocity)  "VIE_EgoVelocity"
  Selector/1 -> HWA_RightLane/1(Object_VX)
  Selector1/1 -> HWA_RightLane/2(Object_VY)
  Selector2/1 -> HWA_RightLane/3(object_MovingState)
  Selector3/1 -> HWA_RightLane/4(PP_ObjMovingDirSignalProcessing)
  Selector4/1 -> HWA_RightLane/5(Object_HeadingAngle)
  Selector5/1 -> HWA_RightLane/6(Object_Type)
  Selector6/1 -> HWA_RightLane/7(TOS_TLJ_RightLaneConfirm_Flag)
  Selector7/1 -> HWA_RightLane/8(Object_DX)
  Selector8/1 -> HWA_RightLane/10(Object_Fus_Type)
  Selector9/1 -> HWA_RightLane/11(PP_ObjFusType_FC_FR_Confirm)
  Selector10/1 -> HWA_RightLane/12(PP_ObjFusType_FR_Confirm)
  Selector11/1 -> HWA_RightLane/13(PP_ObjFusType_FC_Confirm)
  object_MovingState/1 -> Selector2/1  "object_MovingState"
  PP_ObjFusType_FC_Confirm/1 -> Selector11/1  "PP_ObjFusType_FC_Confirm"
  PP_ObjFusType_FR_Confirm/1 -> Selector10/1  "PP_ObjFusType_FR_Confirm"
  PP_ObjFusType_FC_FR_Confirm/1 -> Selector9/1  "PP_ObjFusType_FC_FR_Confirm"
  Object_Fus_Type/1 -> Selector8/1  "Object_Fus_Type"
  Object_DX/1 -> Selector7/1  "Object_DX"
  TOS_TLJ_RightLaneConfirm_Flag/1 -> Selector6/1  "TOS_TLJ_RightLaneConfirm_Flag"
  Object_Type/1 -> Selector5/1  "Object_Type"
  Object_VY/1 -> Selector1/1  "Object_VY"
  Object_VX/1 -> Selector/1  "Object_VX"
  PP_ObjMovingDirSignalProcessing/1 -> Selector3/1  "PP_ObjMovingDirSignalProcessing"
  Object_HeadingAngle/1 -> Selector4/1  "Object_HeadingAngle"
  HWA_RightLane_ObjIndex/1 -> Selector/2, Selector1/2, Selector12/2, Selector11/2, Selector10/2, Selector9/2, Selector8/2, Selector7/2, Selector6/2, Selector5/2, Selector4/2, Selector3/2, Selector2/2  "HWA_RightLane_ObjIndex"
  Object_DY/1 -> Selector12/1  "Object_DX"
  Selector12/1 -> HWA_RightLane/9(Object_DY)
  HWA_RightLane/1(TOS_HWA_TargetInRightLane_b) -> TOS_HWA_TargetInRightLane_b/1
  HWA_RightLane/11(TOS_HWA_RightRear_DyConfirm_ObserVale) -> TOS_HWA_RightRear_DyConfirm_ObserVale/1
  HWA_RightLane/2(TOS_HWA_RightFront_TargConfirm_b) -> TOS_HWA_RightFront_TargConfirm_b/1
  HWA_RightLane/3(TOS_HWA_RightRear_TargConfirm_b) -> TOS_HWA_RightRear_TargConfirm_b/1
  HWA_RightLane/4(TOS_HWA_RightFront_FusType_ObserVale) -> TOS_HWA_RightFront_FusType_ObserVale/1
  HWA_RightLane/5(TOS_HWA_InRightLane_Front_Flag_ObserVale) -> TOS_HWA_InRightLane_Front_Flag_ObserVale/1
  HWA_RightLane/6(TOS_HWA_RightFront_TargMovDir_ObserVale) -> TOS_HWA_RightFront_TargMovDir_ObserVale/1
  HWA_RightLane/7(TOS_HWA_RightRear_MovState_ObserVale) -> TOS_HWA_RightRear_MovState_ObserVale/1
  HWA_RightLane/8(TOS_HWA_RightRear_FusionType_ObserVale) -> TOS_HWA_RightRear_FusionType_ObserVale/1
  HWA_RightLane/9(TOS_HWA_InRightLane_Rear_Flag_ObserVale) -> TOS_HWA_InRightLane_Rear_Flag_ObserVale/1
  HWA_RightLane/10(TOS_HWA_RightRear_TargetMovingDir_ObserVale) -> TOS_HWA_RightRear_TargetMovingDir_ObserVale/1

== system PubIfDecisionTOS_MDL/TOS_20201112/TOS_2012080320/TOS/LC_LCKie_ELK/TOS_HWA/RightLane/TOS_HWA_RightLane/TOS_HWA_RightLane/TOS_HWA_Default ==
  Action Port : ActionPort  ActionPortLabel=if(u1 ~= 0)
  Constant{1..11} (11 alike) : Constant  Value=0  OutDataTypeStr=boolean
  TOS_HWA_TargetInRightLane_b : Outport
  TOS_HWA_RightFront_TargConfirm_b : Outport  Port=2
  TOS_HWA_RightRear_TargConfirm_b : Outport  Port=3
  TOS_HWA_RightFront_FusType_ObserVale : Outport  Port=4
  TOS_HWA_InRightLane_Front_Flag_ObserVale : Outport  Port=5
  TOS_HWA_RightFront_TargMovDir_ObserVale : Outport  Port=6
  TOS_HWA_RightRear_MovState_ObserVale : Outport  Port=7
  TOS_HWA_RightRear_FusionType_ObserVale : Outport  Port=8
  TOS_HWA_InRightLane_Rear_Flag_ObserVale : Outport  Port=9
  TOS_HWA_RightRear_TargetMovingDir_ObserVale : Outport  Port=10
  TOS_HWA_RightRear_DyConfirm_ObserVale : Outport  Port=11
  wires:
  Constant4/1 -> TOS_HWA_TargetInRightLane_b/1
  Constant1/1 -> TOS_HWA_RightFront_TargConfirm_b/1
  Constant2/1 -> TOS_HWA_RightFront_FusType_ObserVale/1
  Constant3/1 -> TOS_HWA_RightRear_TargConfirm_b/1
  Constant7/1 -> TOS_HWA_RightRear_MovState_ObserVale/1
  Constant6/1 -> TOS_HWA_RightRear_FusionType_ObserVale/1
  Constant5/1 -> TOS_HWA_RightFront_TargMovDir_ObserVale/1
  Constant8/1 -> TOS_HWA_InRightLane_Front_Flag_ObserVale/1
  Constant9/1 -> TOS_HWA_InRightLane_Rear_Flag_ObserVale/1
  Constant10/1 -> TOS_HWA_RightRear_DyConfirm_ObserVale/1
  Constant11/1 -> TOS_HWA_RightRear_TargetMovingDir_ObserVale/1

== system PubIfDecisionTOS_MDL/TOS_20201112/TOS_2012080320/TOS/P0_Trajectory_V1.0/CordinatConvert/CordinatConvert/CordinatConvert/TrackRecord_CordinatConvert/CordinatConvertDefault ==
  Action Port : ActionPort  ActionPortLabel=if(u1 == 1)
  Constant : Constant  Value=single(0)
  Constant1 : Constant  Value=single(0)
  Constant2 : Constant  Value=uint32(0)
  Constant3 : Constant  Value=uint8(0)
  P0_dx_TrackRecord_CordinatConvert_K1 : Outport
  P0_dy_TrackRecord_CordinatConvert_K1 : Outport  Port=2
  P0_Counter_TrackRecord_CordinatConvert_K1 : Outport  Port=3
  P0_ID_TrackRecord_CordinatConvert_K1 : Outport  Port=4
  wires:
  Constant/1 -> P0_dx_TrackRecord_CordinatConvert_K1/1
  Constant1/1 -> P0_dy_TrackRecord_CordinatConvert_K1/1
  Constant2/1 -> P0_Counter_TrackRecord_CordinatConvert_K1/1
  Constant3/1 -> P0_ID_TrackRecord_CordinatConvert_K1/1

== system PubIfDecisionTOS_MDL/TOS_20201112/TOS_2012080320/TOS/P0_Trajectory_V1.0/CordinatConvert/CordinatConvert/CordinatConvert/TrackRecord_CordinatConvert/TrackRecord_CordinatConvert ==
  EgoVeh_OffsetX : Inport
  EgoVeh_OffsetY : Inport  Port=2
  EgoVeh_OffsetAngle : Inport  Port=3
  P0_dx_TrackRecord_K1 : Inport  Port=4
  P0_dy_TrackRecord_K1 : Inport  Port=5
  P0_Counter_TrackRecord : Inport  Port=6
  P0_ID_TrackRecord_K1 : Inport  Port=7
  Action Port : ActionPort  ActionPortLabel=else
  Add : Sum
  Product{,1..3} (4 alike) : Product
  Signal Copy : SignalConversion  OverrideOpt=off
  Signal Copy1 : SignalConversion  OverrideOpt=off
  Sin : Trigonometry
  Sin1 : Trigonometry  Operator=cos
  Subtract : Sum  Inputs=+-
  Subtract1 : Sum  Inputs=+-
  Subtract2 : Sum  Inputs=+-
  P0_dx_TrackRecord_CordinatConvert_K1 : Outport
  P0_dy_TrackRecord_CordinatConvert_K1 : Outport  Port=2
  P0_Counter_TrackRecord_CordinatConvert_K1 : Outport  Port=3
  P0_ID_TrackRecord_CordinatConvert_K2 : Outport  Port=4
  wires:
  Signal Copy/1 -> P0_Counter_TrackRecord_CordinatConvert_K1/1
  P0_Counter_TrackRecord/1 -> Signal Copy/1
  Subtract2/1 -> P0_dx_TrackRecord_CordinatConvert_K1/1
  EgoVeh_OffsetX/1 -> Subtract/2
  EgoVeh_OffsetY/1 -> Subtract1/2
  P0_dx_TrackRecord_K1/1 -> Subtract/1
  Add/1 -> P0_dy_TrackRecord_CordinatConvert_K1/1
  Product3/1 -> Add/2
  Subtract/1 -> Product/1, Product2/1
  Sin/1 -> Product1/2, Product2/2
  EgoVeh_OffsetAngle/1 -> Sin1/1, Sin/1
  P0_dy_TrackRecord_K1/1 -> Subtract1/1
  Product1/1 -> Subtract2/2
  Product/1 -> Subtract2/1
  Product2/1 -> Add/1
  Sin1/1 -> Product/2, Product3/2
  Subtract1/1 -> Product1/1, Product3/1
  P0_ID_TrackRecord_K1/1 -> Signal Copy1/1
  Signal Copy1/1 -> P0_ID_TrackRecord_CordinatConvert_K2/1

== system PubIfDecisionTOS_MDL/TOS_20201112/TOS_2012080320/TOS/P0_Trajectory_V1.0/CordinatConvert/CordinatConvert1/CordinatConvert/TrackRecord_CordinatConvert/CordinatConvertDefault ==
  Action Port : ActionPort
  Constant : Constant  Value=single(0)
  Constant1 : Constant  Value=single(0)
  Constant2 : Constant  Value=uint32(0)
  Constant3 : Constant  Value=uint8(0)
  P0_dx_TrackRecord_CordinatConvert_K1 : Outport
  P0_dy_TrackRecord_CordinatConvert_K1 : Outport  Port=2
  P0_Counter_TrackRecord_CordinatConvert_K1 : Outport  Port=3
  P0_ID_TrackRecord_CordinatConvert_K1 : Outport  Port=4
  wires:
  Constant3/1 -> P0_ID_TrackRecord_CordinatConvert_K1/1
  Constant2/1 -> P0_Counter_TrackRecord_CordinatConvert_K1/1
  Constant1/1 -> P0_dy_TrackRecord_CordinatConvert_K1/1
  Constant/1 -> P0_dx_TrackRecord_CordinatConvert_K1/1

== system PubIfDecisionTOS_MDL/TOS_20201112/TOS_2012080320/TOS/P0_Trajectory_V1.0/CordinatConvert/CordinatConvert1/CordinatConvert/TrackRecord_CordinatConvert/TrackRecord_CordinatConvert ==
  EgoVeh_OffsetX : Inport
  EgoVeh_OffsetY : Inport  Port=2
  EgoVeh_OffsetAngle : Inport  Port=3
  P0_dx_TrackRecord_K1 : Inport  Port=4
  P0_dy_TrackRecord_K1 : Inport  Port=5
  P0_Counter_TrackRecord : Inport  Port=6
  P0_ID_TrackRecord_K1 : Inport  Port=7
  Action Port : ActionPort
  Add : Sum
  Product{,1..3} (4 alike) : Product
  Signal Copy : SignalConversion  OverrideOpt=off
  Signal Copy1 : SignalConversion  OverrideOpt=off
  Sin : Trigonometry
  Sin1 : Trigonometry  Operator=cos
  Subtract : Sum  Inputs=+-
  Subtract1 : Sum  Inputs=+-
  Subtract2 : Sum  Inputs=+-
  P0_dx_TrackRecord_CordinatConvert_K1 : Outport
  P0_dy_TrackRecord_CordinatConvert_K1 : Outport  Port=2
  P0_Counter_TrackRecord_CordinatConvert_K1 : Outport  Port=3
  P0_ID_TrackRecord_CordinatConvert_K2 : Outport  Port=4
  wires:
  Signal Copy1/1 -> P0_ID_TrackRecord_CordinatConvert_K2/1
  P0_ID_TrackRecord_K1/1 -> Signal Copy1/1
  Subtract1/1 -> Product3/1, Product1/1
  Sin1/1 -> Product3/2, Product/2
  Product2/1 -> Add/1
  Product/1 -> Subtract2/1
  Product1/1 -> Subtract2/2
  P0_dy_TrackRecord_K1/1 -> Subtract1/1
  EgoVeh_OffsetAngle/1 -> Sin/1, Sin1/1
  Sin/1 -> Product2/2, Product1/2
  Subtract/1 -> Product2/1, Product/1
  Product3/1 -> Add/2
  Add/1 -> P0_dy_TrackRecord_CordinatConvert_K1/1
  P0_dx_TrackRecord_K1/1 -> Subtract/1
  EgoVeh_OffsetY/1 -> Subtract1/2
  EgoVeh_OffsetX/1 -> Subtract/2
  Subtract2/1 -> P0_dx_TrackRecord_CordinatConvert_K1/1
  P0_Counter_TrackRecord/1 -> Signal Copy/1
  Signal Copy/1 -> P0_Counter_TrackRecord_CordinatConvert_K1/1

== system PubIfDecisionTOS_MDL/TOS_20201112/TOS_2012080320/PIL_1029/ObjCutInOut_Prob/ObjectCutIn/CutInProb_Calculate/CutInProb_Calculate_/CutInPredictDis_dy/CutInPredictTime/CarTruck_ToCenterLine_dy_Predict ==
  ObjectType : Inport
  PP_ObjectToCenterLine_vyc : Inport  Port=2  OutDataTypeStr=single
  Abs : Abs
  Compare To Constant : simulink/Logic and Bit Operations/Compare To Constant  relop===  const=OFM_OBJ_TYPE_E.CAR  OutDataTypeStr=boolean
      settings: AttributesFormatString=OFM_OBJ_TYPE_E.CAR = 2
  Compare To Constant1 : simulink/Logic and Bit Operations/Compare To Constant  relop===  const=OFM_OBJ_TYPE_E.TRUCK  OutDataTypeStr=boolean
      settings: AttributesFormatString=OFM_OBJ_TYPE_E.TRUCK = 3
  Compare To Constant2 : simulink/Logic and Bit Operations/Compare To Constant  relop=>  const=P_TOS_CutinObjvyThre_CarTruck_Val  OutDataTypeStr=boolean
      settings: AttributesFormatString=P_TOS_CutinObjvyThre_CarTruck_Val = 0.06
  Data Type Conversion : DataTypeConversion  OutDataTypeStr=Enum: OFM_OBJ_TYPE_E
  Logical Operator1 : Logic  AllPortsSameDT=off  OutDataTypeStr=boolean
  Logical Operator16 : Logic  Operator=OR  AllPortsSameDT=off  OutDataTypeStr=boolean
  CarTruck_ToCenterLine_dy_Predict : Outport
  wires:
  ObjectType/1 -> Data Type Conversion/1
  Logical Operator16/1 -> Logical Operator1/1
  Compare To Constant1/1 -> Logical Operator16/2
  Data Type Conversion/1 -> Compare To Constant1/1, Compare To Constant/1
  Compare To Constant/1 -> Logical Operator16/1
  PP_ObjectToCenterLine_vyc/1 -> Abs/1
  Compare To Constant2/1 -> Logical Operator1/2
  Abs/1 -> Compare To Constant2/1
  Logical Operator1/1 -> CarTruck_ToCenterLine_dy_Predict/1

== system PubIfDecisionTOS_MDL/TOS_20201112/TOS_2012080320/PIL_1029/ObjCutInOut_Prob/ObjectCutIn/CutInProb_Calculate/CutInProb_Calculate_/CutInPredictDis_dy/CutInPredictTime/ObjectToCenterLine_dy_Predict ==
  note: 目标在中心线右侧
  note: 目标在中心线左侧
  ObjectToCenterLine_dy_Filt : Inport  OutDataTypeStr=single
  ObjectToCenterLine_dy : Inport  Port=2
  Add : Sum  Inputs=+-  OutDataTypeStr=single
  Compare To Constant : simulink/Logic and Bit Operations/Compare To Constant  relop=<  const=C_TOS_ObjToCenterLine_ConstantVal_Zeros  OutDataTypeStr=boolean
      settings: AttributesFormatString=C_TOS_ObjToCenterLine_ConstantVal_Zeros = 0
  Compare To Constant1 : simulink/Logic and Bit Operations/Compare To Constant  relop=<  const=P_TOS_CutIn_ObjectToCenterLine_Rightdy_Con  OutDataTypeStr=boolean
      settings: AttributesFormatString=P_TOS_CutIn_ObjectToCenterLine_Rightdy_Con = -0.1
  Compare To Constant2 : simulink/Logic and Bit Operations/Compare To Constant  relop=>=  const=P_TOS_CutIn_ObjectToCenterLine_Leftdy_Con  OutDataTypeStr=boolean
      settings: AttributesFormatString=P_TOS_CutIn_ObjectToCenterLine_Leftdy_Con = 0.1
  Compare To Constant3 : simulink/Logic and Bit Operations/Compare To Constant  relop=>=  const=C_TOS_ObjToCenterLine_ConstantVal_Zeros  OutDataTypeStr=boolean
      settings: AttributesFormatString=C_TOS_ObjToCenterLine_ConstantVal_Zeros = 0
  Logical Operator : Logic  AllPortsSameDT=off  OutDataTypeStr=boolean
  Logical Operator1 : Logic  Operator=OR  AllPortsSameDT=off  OutDataTypeStr=boolean
  Logical Operator2 : Logic  AllPortsSameDT=off  OutDataTypeStr=boolean
  Out1 : Outport
  wires:
  ObjectToCenterLine_dy/1 -> Add/2, [ObjectToCenterLine_dy]
  ObjectToCenterLine_dy_Filt/1 -> Add/1
  Compare To Constant2/1 -> Logical Operator/1
  Logical Operator/1 -> Logical Operator1/2
  Logical Operator2/1 -> Logical Operator1/1
  Compare To Constant/1 -> Logical Operator2/1
  [ObjectToCenterLine_dy] -> Compare To Constant/1
  Add/1 -> Compare To Constant2/1, Compare To Constant1/1
  Compare To Constant3/1 -> Logical Operator/2
  Compare To Constant1/1 -> Logical Operator2/2
  Logical Operator1/1 -> Out1/1
  [ObjectToCenterLine_dy] -> Compare To Constant3/1

== system PubIfDecisionTOS_MDL/TOS_20201112/TOS_2012080320/PIL_1029/ObjCutInOut_Prob/ObjectCutIn/CutInProb_Calculate/CutInProb_Calculate_/CutInProb/CutInObjWidthConstraint/ObjectWidth_Check ==
  ObjectType : Inport
  Object_Width : Inport  Port=2
  Compare To Constant3 : simulink/Logic and Bit Operations/Compare To Constant  relop===  const=OFM_OBJ_TYPE_E.CAR  OutDataTypeStr=boolean
      settings: AttributesFormatString=OFM_OBJ_TYPE_E.CAR = 2
  Compare To Constant4 : simulink/Logic and Bit Operations/Compare To Constant  relop===  const=OFM_OBJ_TYPE_E.TRUCK  OutDataTypeStr=boolean
      settings: AttributesFormatString=OFM_OBJ_TYPE_E.TRUCK = 3
  Compare To Constant5 : simulink/Logic and Bit Operations/Compare To Constant  relop===  const=OFM_OBJ_TYPE_E.MOTORBIKE  OutDataTypeStr=boolean
      settings: AttributesFormatString=OFM_OBJ_TYPE_E.MOTORBIKE = 4
  Compare To Constant6 : simulink/Logic and Bit Operations/Compare To Constant  relop===  const=OFM_OBJ_TYPE_E.BICYCLE  OutDataTypeStr=boolean
      settings: AttributesFormatString=OFM_OBJ_TYPE_E.BICYCLE = 5
  Compare To Constant7 : simulink/Logic and Bit Operations/Compare To Constant  relop===  const=OFM_OBJ_TYPE_E.PEDESTRIAN  OutDataTypeStr=boolean
      settings: AttributesFormatString=OFM_OBJ_TYPE_E.PEDESTRIAN = 6
  Data Type Conversion1 : DataTypeConversion  OutDataTypeStr=Enum: OFM_OBJ_TYPE_E
  Logical Operator1 : Logic  Operator=OR  AllPortsSameDT=off  OutDataTypeStr=boolean
  Logical Operator2 : Logic  Operator=OR  AllPortsSameDT=off  OutDataTypeStr=boolean
  Saturation1 : Saturate  UpperLimit=2.0  LowerLimit=1.65
  Saturation2 : Saturate  UpperLimit=0.8  LowerLimit=0.4
  Saturation3 : Saturate  LowerLimit=0.5
  Switch2 : Switch  Criteria=u2 ~= 0
  Switch3 : Switch  Criteria=u2 ~= 0
  Switch4 : Switch  Criteria=u2 ~= 0
  ObjectWidth : Outport
  wires:
  Object_Width/1 -> Saturation2/1, Switch4/3, Saturation3/1, Saturation1/1
  Compare To Constant5/1 -> Logical Operator2/1
  Saturation3/1 -> Switch4/1
  Compare To Constant3/1 -> Logical Operator1/1
  ObjectType/1 -> Data Type Conversion1/1
  Compare To Constant7/1 -> Switch4/2
  Logical Operator2/1 -> Switch3/2
  Compare To Constant6/1 -> Logical Operator2/2
  Compare To Constant4/1 -> Logical Operator1/2
  Logical Operator1/1 -> Switch2/2
  Saturation1/1 -> Switch2/1
  Data Type Conversion1/1 -> Compare To Constant7/1, Compare To Constant6/1, Compare To Constant5/1, Compare To Constant4/1, Compare To Constant3/1
  Switch4/1 -> Switch3/3
  Saturation2/1 -> Switch3/1
  Switch3/1 -> Switch2/3
  Switch2/1 -> ObjectWidth/1

== system PubIfDecisionTOS_MDL/TOS_20201112/TOS_2012080320/PIL_1029/ObjCutInOut_Prob/ObjectCutIn/CutInProb_Calculate/CutInProb_Calculate_/CutInProb_ScopeConstraint1/ObjectCutinMind1/CutInObjCutoutMov ==
  note: 目标在中心线左侧，向左运动
  note: 目标在中心线右侧，向右运动
  PP_ObjectToCenterLine_vyc : Inport
  ObjectToCenterLine_dy : Inport  Port=2  OutDataTypeStr=single
  Compare To Constant1 : simulink/Logic and Bit Operations/Compare To Constant  relop=>  const=C_TOS_ObjToCenterLine_ConstantVal_Zeros  OutDataTypeStr=boolean
      settings: AttributesFormatString=C_TOS_ObjToCenterLine_ConstantVal_Zeros = 0
  Compare To Constant2 : simulink/Logic and Bit Operations/Compare To Constant  relop=>  const=P_TOS_CutoutObjvyThre_Val  OutDataTypeStr=boolean
      settings: AttributesFormatString=P_TOS_CutoutObjvyThre_Val = 0.1
  Compare To Constant3 : simulink/Logic and Bit Operations/Compare To Constant  relop=<  const=P_TOS_CutoutObjvyThre_NegativeVal  OutDataTypeStr=boolean
      settings: AttributesFormatString=P_TOS_CutoutObjvyThre_NegativeVal = -0.1
  Switch : Switch  Criteria=u2 ~= 0  OutDataTypeStr=single
  CutInObjCutoutMovflg : Outport
  wires:
  Switch/1 -> CutInObjCutoutMovflg/1
  ObjectToCenterLine_dy/1 -> Compare To Constant1/1
  Compare To Constant1/1 -> Switch/2
  PP_ObjectToCenterLine_vyc/1 -> Compare To Constant3/1, Compare To Constant2/1
  Compare To Constant3/1 -> Switch/3
  Compare To Constant2/1 -> Switch/1
